simulink model "sf_pwd"  (Simulink 8.3)
settings: Solver=FixedStepDiscrete  StartTime=0.0  StopTime=Inf  RelTol=1e-3
libraries: simulink x1
settings Model: Creator=pit  LastModifiedBy=eruffaldi
settings OptimizationCC: ExpressionDepthLimit=2147483647  InitFltsAndDblsToZero=on
settings DebuggingCC: FcnCallInpInsideContextMsg=UseLocalSettings
settings SFSimCC: SimParseCustomCode=off

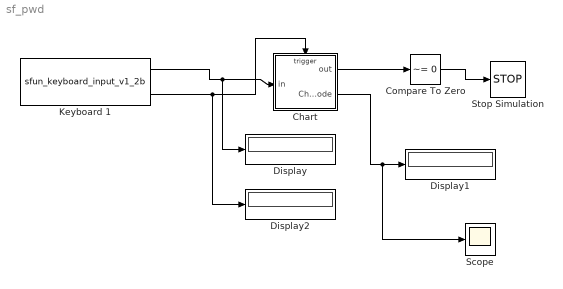
== system sf_pwd ==
  Chart : Stateflow chart  TreatAsAtomicUnit=on
  Compare To Zero : simulink/Logic and Bit Operations/Compare To Zero  relop=~=  OutDataTypeStr=boolean  ZeroCross=off
  Display : Display
  Display1 : Display
  Display2 : Display
  Keyboard 1 : M-S-Function  FunctionName=sfun_keyboard_input_v1_2b  mask(Keyboard Input){}
      mask help: Keyboard Input
      mask Display: fprintf('Keyboard');
  Scope : Scope
  Stop Simulation : Stop
  wires:
  Keyboard 1/1 -> Display/1, Chart/1(in)
  Chart/1(out) -> Compare To Zero/1
  Compare To Zero/1 -> Stop Simulation/1
  Keyboard 1/2 -> Display2/1, Chart/Trigger
  Chart/2(ChartMode) -> Scope/1, Display1/1

== stateflow chart Chart ==
  state s0
    entry: out=0
  state s01
  state s02
  state s03
  state s04
    entry: out=1
  (default) -> s0
  s03 -> s04 [order 1] : [in==52]
  s02 -> s03 [order 1] : [in==49]
  s01 -> s02 [order 1] : [in==52]
  s0 -> s01 : [in==48]
  s04 -> s0
  s03 -> s0 [order 2]
  s02 -> s0 [order 2]
  s01 -> s0 [order 2]
  data: in input double; out output double; ChartMode output Enum: ChartModeType
  events: event input RISING_EDGE_EVENT
